simulink model "Ex0_1"  (R2019a)
settings: Solver=VariableStepAuto  StartTime=0.0  StopTime=10.0  RelTol=1e-3
values from neighbouring files (symbols this model uses):
  K1 = 1    [value0.m]    (also in value1.m = 0.5)
  K2 = 2    [value0.m]    (also in value1.m = 1)
  K3 = 3    [value0.m]    (also in value1.m = 2)
  T = 1    [value0.m]    (also in value1.m = 2)
settings Model: Creator=Takumi SHIOTA  LastModifiedBy=Takumi SHIOTA

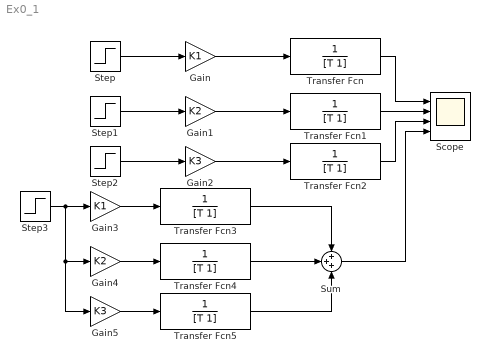
== system Ex0_1 ==
  Gain : Gain  Gain=K1
  Gain1 : Gain  Gain=K2
  Gain2 : Gain  Gain=K3
  Gain3 : Gain  Gain=K1
  Gain4 : Gain  Gain=K2
  Gain5 : Gain  Gain=K3
  Scope : Scope  NumInputPorts=4
  Step{,1..3} (4 alike) : Step  SampleTime=0
  Sum : Sum  Inputs=+++
  Transfer Fcn{,1..5} (6 alike) : TransferFcn  Denominator=[T 1]
  wires:
  Step2/1 -> Gain2/1
  Step1/1 -> Gain1/1
  Transfer Fcn1/1 -> Scope/2
  Gain1/1 -> Transfer Fcn1/1
  Gain/1 -> Transfer Fcn/1
  Transfer Fcn2/1 -> Scope/3
  Gain3/1 -> Transfer Fcn3/1
  Step/1 -> Gain/1
  Gain4/1 -> Transfer Fcn4/1
  Transfer Fcn/1 -> Scope/1
  Transfer Fcn3/1 -> Sum/1
  Transfer Fcn4/1 -> Sum/2
  Gain5/1 -> Transfer Fcn5/1
  Transfer Fcn5/1 -> Sum/3
  Gain2/1 -> Transfer Fcn2/1
  Sum/1 -> Scope/4
  Step3/1 -> Gain5/1, Gain4/1, Gain3/1
